simulink model "IOT_Charger"  (R2024b)
settings: Solver=ode23tb  StartTime=0.0  StopTime=1  RelTol=1e-3  EnableMultiTasking=on
PreLoadFcn:
  | % Data of Solar Panel
  | %5000[W]/130[W]
  | % Total power generated by solar panel reaches 5[KW].
  | % each solar panel generates power 130[kW].
  | V = [0    40 80 120 160 180 200 217 240 260 280];
  | I = 5000/130*[0.68 0.675 0.67 0.665 0.660 0.655 0.640 0.6 0.48 0.28 0];
  | 
  | %subplot(211);plot(V,I);xlabel('Voltage[V]');ylabel('Current[a]')
  | %subplot(212);plot(V.*I);title('Power[W]')
  | 
  | % Sample Time[s]
  | Ts =5e-6;
  | 
  | 
  | %MPPT + PV Control
  | % PI control pamameter of Voltage control(Outer loop)
  | Kp_V = 50e-3;
  | Ki_V = 10;
  | 
  | % PI Control pamameter of Current control(Inner loop)
  | Kp_I = 25e-3;
  | Ki_I = 10;
  | 
  | % Utility Interconnection Control
  | % PI Control pamameter of Voltage control(Outer loop)
  | Kp_V2 = 0.01;
  | Ki_V2 = 25;
  | 
  | % PI control pamameter of Current control(Inner loop)
  | Kp_I2 = 0.01;
  | Ki_I2 = 25;
  | 
  | 
  | % Difference of voltege using in MPPT
  | dV = 0.5;
  | 
  | % Battery Control
  | % PI Control pamameter of Voltage control(Outer loop)
  | Kp_VB = 0.4;
  | Ki_VB = 2;
  | 
  | % PI control pamameter of Current control(Inner loop)
  | Kp_IB = 0.1;
  | Ki_IB = 0.5;
undefined symbols (not defined in the file): Ion, Lithium, sigbuilder_block
libraries: spsBreakerLib x120, spsSeriesRLCBranchLib x72, spsBatteryLib x43, spsIdealSwitchLib x29, spsVoltageMeasurementLib x25, spsMosfetLib x19, slpidlib x17, spsSeriesRLCLoadLib x12, spsPWMGeneratorDCDCLib x11, spsCurrentMeasurementLib x10, spsDiodeLib x6, spsPWMGenerator2LevelLib x5
(part 4 of 6)

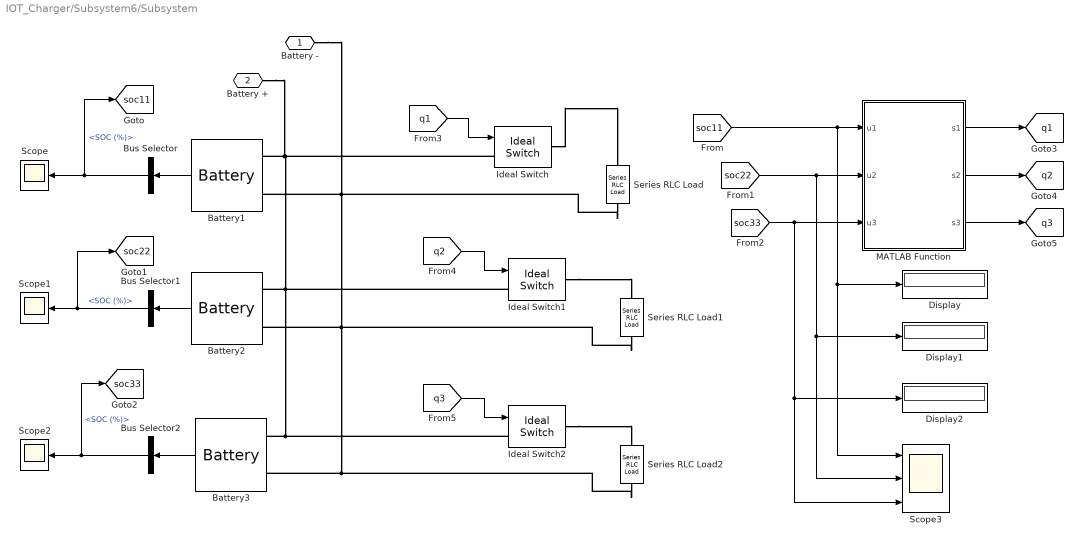
== system IOT_Charger/Subsystem6/Subsystem ==
  Battery1 : spsBatteryLib/Battery  BatType=Lithium-Ion  NomV=3.6  NomQ=4  SOC=100  Batt_Tr=1  PresetModel=on  MaxQ=4  MinV=2.7  FullV=4.1904  Dis_rate=1.7391  R=0.009  Normal_OP=3.6174  expZone="[3.8894     0.19652]"
  Battery2 : spsBatteryLib/Battery  BatType=Lithium-Ion  NomV=3.6  NomQ=4  SOC=60  Batt_Tr=1  PresetModel=on  MaxQ=4  MinV=2.7  FullV=4.1904  Dis_rate=1.7391  R=0.009  Normal_OP=3.6174  expZone="[3.8894     0.19652]"
  Battery3 : spsBatteryLib/Battery  BatType=Lithium-Ion  NomV=3.6  NomQ=4  SOC=30  Batt_Tr=1  PresetModel=on  MaxQ=4  MinV=2.7  FullV=4.1904  Dis_rate=1.7391  R=0.009  Normal_OP=3.6174  expZone="[3.8894     0.19652]"
  Bus Selector : BusSelector  OutputSignals=SOC (%)
  Bus Selector1 : BusSelector  OutputSignals=SOC (%)
  Bus Selector2 : BusSelector  OutputSignals=SOC (%)
  Display : Display
  Display1 : Display
  Display2 : Display
  Ideal Switch : spsIdealSwitchLib/Ideal Switch  Ron=0.001  Lon=0  IC=0  Rs=1e5  Cs=inf  Measurements=off
  Ideal Switch1 : spsIdealSwitchLib/Ideal Switch  Ron=0.001  Lon=0  IC=0  Rs=1e5  Cs=inf  Measurements=off
  Ideal Switch2 : spsIdealSwitchLib/Ideal Switch  Ron=0.001  Lon=0  IC=0  Rs=1e5  Cs=inf  Measurements=off
  MATLAB Function : MATLAB Function  TreatAsAtomicUnit=on
  Scope : Scope
  Scope1 : Scope
  Scope2 : Scope
  Scope3 : Scope  NumInputPorts=3
  Series RLC Load : spsSeriesRLCLoadLib/Series RLC Load  LConnTagsString=a  RConnTagsString=__new0  NominalVoltage=1000  NominalFrequency=60  ActivePower=10e3  InductivePower=0  CapacitivePower=0  Setx0=off  InitialVoltage=0  SetiL0=off  InitialCurrent=0  Measurements=None  LoadType=constant Z
  Series RLC Load1 : spsSeriesRLCLoadLib/Series RLC Load  LConnTagsString=a  RConnTagsString=__new0  NominalVoltage=1000  NominalFrequency=60  ActivePower=10e3  InductivePower=0  CapacitivePower=0  Setx0=off  InitialVoltage=0  SetiL0=off  InitialCurrent=0  Measurements=None  LoadType=constant Z
  Series RLC Load2 : spsSeriesRLCLoadLib/Series RLC Load  LConnTagsString=a  RConnTagsString=__new0  NominalVoltage=1000  NominalFrequency=60  ActivePower=10e3  InductivePower=0  CapacitivePower=0  Setx0=off  InitialVoltage=0  SetiL0=off  InitialCurrent=0  Measurements=None  LoadType=constant Z
  Battery - : PMIOPort  Side=Left
  Battery + : PMIOPort  Port=2  Side=Left
  tag scope: q1=global, q2=global, q3=global, soc11=global, soc22=global, soc33=global
  wires:
  Battery2/1 -> Bus Selector1/1
  Bus Selector/1 -> [soc11], Scope/1  "<SOC (%)>"
  [q3] -> Ideal Switch2/1
  Bus Selector2/1 -> [soc33], Scope2/1  "<SOC (%)>"
  Bus Selector1/1 -> [soc22], Scope1/1  "<SOC (%)>"
  Battery3/1 -> Bus Selector2/1
  [soc22] -> MATLAB Function/2(u2), Display1/1, Scope3/2
  [soc11] -> Display/1, Scope3/1, MATLAB Function/1(u1)
  Battery1/1 -> Bus Selector/1
  [soc33] -> Display2/1, Scope3/3, MATLAB Function/3(u3)
  MATLAB Function/2(s2) -> [q2]
  MATLAB Function/3(s3) -> [q3]
  MATLAB Function/1(s1) -> [q1]
  [q1] -> Ideal Switch/1
  [q2] -> Ideal Switch1/1
  connections:
  Series RLC Load/RConn1 -- Battery3/LConn2 -- Series RLC Load2/RConn1 -- Battery2/LConn2 -- Series RLC Load1/RConn1 -- Battery -/RConn1 -- Battery1/LConn2
  Ideal Switch1/RConn1 -- Series RLC Load1/LConn1
  Ideal Switch2/RConn1 -- Series RLC Load2/LConn1
  Ideal Switch/RConn1 -- Series RLC Load/LConn1
  Ideal Switch/LConn1 -- Battery +/RConn1 -- Battery1/LConn1 -- Battery3/LConn1 -- Ideal Switch2/LConn1 -- Battery2/LConn1 -- Ideal Switch1/LConn1

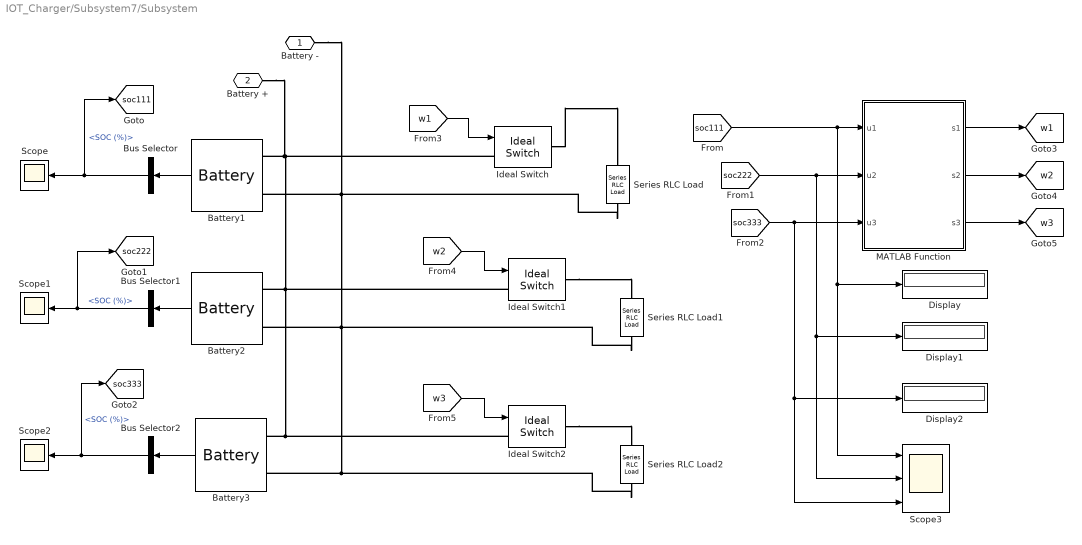
== system IOT_Charger/Subsystem7/Subsystem ==
  Battery1 : spsBatteryLib/Battery  BatType=Lithium-Ion  NomV=3.6  NomQ=4  SOC=100  Batt_Tr=1  PresetModel=on  MaxQ=4  MinV=2.7  FullV=4.1904  Dis_rate=1.7391  R=0.009  Normal_OP=3.6174  expZone="[3.8894     0.19652]"
  Battery2 : spsBatteryLib/Battery  BatType=Lithium-Ion  NomV=3.6  NomQ=4  SOC=60  Batt_Tr=1  PresetModel=on  MaxQ=4  MinV=2.7  FullV=4.1904  Dis_rate=1.7391  R=0.009  Normal_OP=3.6174  expZone="[3.8894     0.19652]"
  Battery3 : spsBatteryLib/Battery  BatType=Lithium-Ion  NomV=3.6  NomQ=4  SOC=30  Batt_Tr=1  PresetModel=on  MaxQ=4  MinV=2.7  FullV=4.1904  Dis_rate=1.7391  R=0.009  Normal_OP=3.6174  expZone="[3.8894     0.19652]"
  Bus Selector : BusSelector  OutputSignals=SOC (%)
  Bus Selector1 : BusSelector  OutputSignals=SOC (%)
  Bus Selector2 : BusSelector  OutputSignals=SOC (%)
  Display : Display
  Display1 : Display
  Display2 : Display
  Ideal Switch : spsIdealSwitchLib/Ideal Switch  Ron=0.001  Lon=0  IC=0  Rs=1e5  Cs=inf  Measurements=off
  Ideal Switch1 : spsIdealSwitchLib/Ideal Switch  Ron=0.001  Lon=0  IC=0  Rs=1e5  Cs=inf  Measurements=off
  Ideal Switch2 : spsIdealSwitchLib/Ideal Switch  Ron=0.001  Lon=0  IC=0  Rs=1e5  Cs=inf  Measurements=off
  MATLAB Function : MATLAB Function  TreatAsAtomicUnit=on
  Scope : Scope
  Scope1 : Scope
  Scope2 : Scope
  Scope3 : Scope  NumInputPorts=3
  Series RLC Load : spsSeriesRLCLoadLib/Series RLC Load  LConnTagsString=a  RConnTagsString=__new0  NominalVoltage=1000  NominalFrequency=60  ActivePower=10e3  InductivePower=0  CapacitivePower=0  Setx0=off  InitialVoltage=0  SetiL0=off  InitialCurrent=0  Measurements=None  LoadType=constant Z
  Series RLC Load1 : spsSeriesRLCLoadLib/Series RLC Load  LConnTagsString=a  RConnTagsString=__new0  NominalVoltage=1000  NominalFrequency=60  ActivePower=10e3  InductivePower=0  CapacitivePower=0  Setx0=off  InitialVoltage=0  SetiL0=off  InitialCurrent=0  Measurements=None  LoadType=constant Z
  Series RLC Load2 : spsSeriesRLCLoadLib/Series RLC Load  LConnTagsString=a  RConnTagsString=__new0  NominalVoltage=1000  NominalFrequency=60  ActivePower=10e3  InductivePower=0  CapacitivePower=0  Setx0=off  InitialVoltage=0  SetiL0=off  InitialCurrent=0  Measurements=None  LoadType=constant Z
  Battery - : PMIOPort  Side=Left
  Battery + : PMIOPort  Port=2  Side=Left
  tag scope: soc111=global, soc222=global, soc333=global, w1=global, w2=global, w3=global
  wires:
  Battery2/1 -> Bus Selector1/1
  Bus Selector/1 -> [soc111], Scope/1  "<SOC (%)>"
  [w3] -> Ideal Switch2/1
  Bus Selector2/1 -> [soc333], Scope2/1  "<SOC (%)>"
  Bus Selector1/1 -> [soc222], Scope1/1  "<SOC (%)>"
  Battery3/1 -> Bus Selector2/1
  [soc222] -> MATLAB Function/2(u2), Display1/1, Scope3/2
  [soc111] -> Display/1, Scope3/1, MATLAB Function/1(u1)
  Battery1/1 -> Bus Selector/1
  [soc333] -> Display2/1, Scope3/3, MATLAB Function/3(u3)
  MATLAB Function/2(s2) -> [w2]
  MATLAB Function/3(s3) -> [w3]
  MATLAB Function/1(s1) -> [w1]
  [w1] -> Ideal Switch/1
  [w2] -> Ideal Switch1/1
  connections:
  Series RLC Load/RConn1 -- Battery3/LConn2 -- Series RLC Load2/RConn1 -- Battery2/LConn2 -- Series RLC Load1/RConn1 -- Battery -/RConn1 -- Battery1/LConn2
  Ideal Switch1/RConn1 -- Series RLC Load1/LConn1
  Ideal Switch2/RConn1 -- Series RLC Load2/LConn1
  Ideal Switch/RConn1 -- Series RLC Load/LConn1
  Ideal Switch/LConn1 -- Battery +/RConn1 -- Battery1/LConn1 -- Battery3/LConn1 -- Ideal Switch2/LConn1 -- Battery2/LConn1 -- Ideal Switch1/LConn1

== system IOT_Charger/Vechicle BMS Monitoring/BMS Discharge ==
  Terminal voltage : Inport
  Temperature : Inport  Port=2
  Current : Inport  Port=3
  Constant : Constant  Value=0
  Function logic block : Subsystem
  Switch : Switch  Criteria=u2 ~= 0  SaturateOnIntegerOverflow=off  InputSameDT=off
  Discharge current : Outport
  wires:
  Terminal voltage/1 -> Function logic block/1(Terminal voltage)
  Current/1 -> Switch/3, Function logic block/2(Current)
  Temperature/1 -> Function logic block/3(Temperature)
  Function logic block/1(Discharge Terget) -> Switch/2
  Constant/1 -> Switch/1
  Switch/1 -> Discharge current/1

== system IOT_Charger/Vechicle BMS Monitoring1/BMS Discharge ==
  Terminal voltage : Inport
  Temperature : Inport  Port=2
  Current : Inport  Port=3
  Constant : Constant  Value=0
  Function logic block : Subsystem
  Switch : Switch  Criteria=u2 ~= 0  SaturateOnIntegerOverflow=off  InputSameDT=off
  Discharge current : Outport
  wires:
  Terminal voltage/1 -> Function logic block/1(Terminal voltage)
  Current/1 -> Switch/3, Function logic block/2(Current)
  Temperature/1 -> Function logic block/3(Temperature)
  Function logic block/1(Discharge Terget) -> Switch/2
  Constant/1 -> Switch/1
  Switch/1 -> Discharge current/1

== system IOT_Charger/Vechicle BMS Monitoring2/BMS Discharge ==
  Terminal voltage : Inport
  Temperature : Inport  Port=2
  Current : Inport  Port=3
  Constant : Constant  Value=0
  Function logic block : Subsystem
  Switch : Switch  Criteria=u2 ~= 0  SaturateOnIntegerOverflow=off  InputSameDT=off
  Discharge current : Outport
  wires:
  Terminal voltage/1 -> Function logic block/1(Terminal voltage)
  Current/1 -> Switch/3, Function logic block/2(Current)
  Temperature/1 -> Function logic block/3(Temperature)
  Function logic block/1(Discharge Terget) -> Switch/2
  Constant/1 -> Switch/1
  Switch/1 -> Discharge current/1

== system IOT_Charger/Vechicle BMS Monitoring3/BMS Discharge ==
  Terminal voltage : Inport
  Temperature : Inport  Port=2
  Current : Inport  Port=3
  Constant : Constant  Value=0
  Function logic block : Subsystem
  Switch : Switch  Criteria=u2 ~= 0  SaturateOnIntegerOverflow=off  InputSameDT=off
  Discharge current : Outport
  wires:
  Terminal voltage/1 -> Function logic block/1(Terminal voltage)
  Current/1 -> Switch/3, Function logic block/2(Current)
  Temperature/1 -> Function logic block/3(Temperature)
  Function logic block/1(Discharge Terget) -> Switch/2
  Constant/1 -> Switch/1
  Switch/1 -> Discharge current/1

== system IOT_Charger/Fast charging controller/Fast charging Switching controller/g1 ==
  Constant1 : Constant  Value=0
  Constant2 : Constant
  Display2 : Display
  Display3 : Display
  Switch : Switch  Threshold=150  SaturateOnIntegerOverflow=off  InputSameDT=off
  tag scope: gg1=global
  wires:
  [FS] -> Display3/1, Switch/2
  Switch/1 -> Display2/1, [gg1]
  Constant1/1 -> Switch/3
  Constant2/1 -> Switch/1

== system IOT_Charger/Fast charging controller/Fast charging Switching controller/g2 ==
  Constant1 : Constant  Value=0
  Constant2 : Constant
  Display2 : Display
  Display3 : Display
  Switch : Switch  Threshold=150  SaturateOnIntegerOverflow=off  InputSameDT=off
  tag scope: gg2=global
  wires:
  [FS] -> Display3/1, Switch/2
  Switch/1 -> Display2/1, [gg2]
  Constant1/1 -> Switch/3
  Constant2/1 -> Switch/1

== system IOT_Charger/Fast charging controller/Fast charging Switching controller/g3 ==
  Constant1 : Constant  Value=0
  Constant2 : Constant
  Display2 : Display
  Display3 : Display
  Switch : Switch  Threshold=150  SaturateOnIntegerOverflow=off  InputSameDT=off
  tag scope: gg3=global
  wires:
  [FS] -> Display3/1, Switch/2
  Switch/1 -> Display2/1, [gg3]
  Constant1/1 -> Switch/3
  Constant2/1 -> Switch/1

== system IOT_Charger/Fast charging controller/Fast charging Switching controller/g4 ==
  Constant1 : Constant  Value=0
  Constant2 : Constant
  Display2 : Display
  Display3 : Display
  Switch : Switch  Threshold=150  SaturateOnIntegerOverflow=off  InputSameDT=off
  tag scope: gg4=global
  wires:
  [FS] -> Display3/1, Switch/2
  Switch/1 -> Display2/1, [gg4]
  Constant1/1 -> Switch/3
  Constant2/1 -> Switch/1

== system IOT_Charger/Grid/Wall charger Connection Box/Battery Switching Control ==
  Control : Inport
  Ideal Switch{,1,3..4} (4 alike) : spsIdealSwitchLib/Ideal Switch  Ron=0.001  Lon=0  IC=0  Rs=1e5  Cs=inf  Measurements=off
  NOT : Logic  Operator=NOT  IconShape=distinctive  AllPortsSameDT=off  OutDataTypeStr=boolean
  discharge + : PMIOPort  Side=Left
  discharge - : PMIOPort  Port=2  Side=Left
  charge + : PMIOPort  Port=3  Side=Left
  charge - : PMIOPort  Port=4  Side=Left
  battery + : PMIOPort  Port=5  Side=Right
  battery - : PMIOPort  Port=6  Side=Right
  wires:
  Control/1 -> NOT/1, Ideal Switch1/1, Ideal Switch/1
  NOT/1 -> Ideal Switch4/1, Ideal Switch3/1
  connections:
  charge -/RConn1 -- Ideal Switch4/RConn1
  discharge +/RConn1 -- Ideal Switch/RConn1
  Ideal Switch1/LConn1 -- battery -/RConn1 -- Ideal Switch4/LConn1
  discharge -/RConn1 -- Ideal Switch1/RConn1
  Ideal Switch/LConn1 -- battery +/RConn1 -- Ideal Switch3/LConn1
  charge +/RConn1 -- Ideal Switch3/RConn1

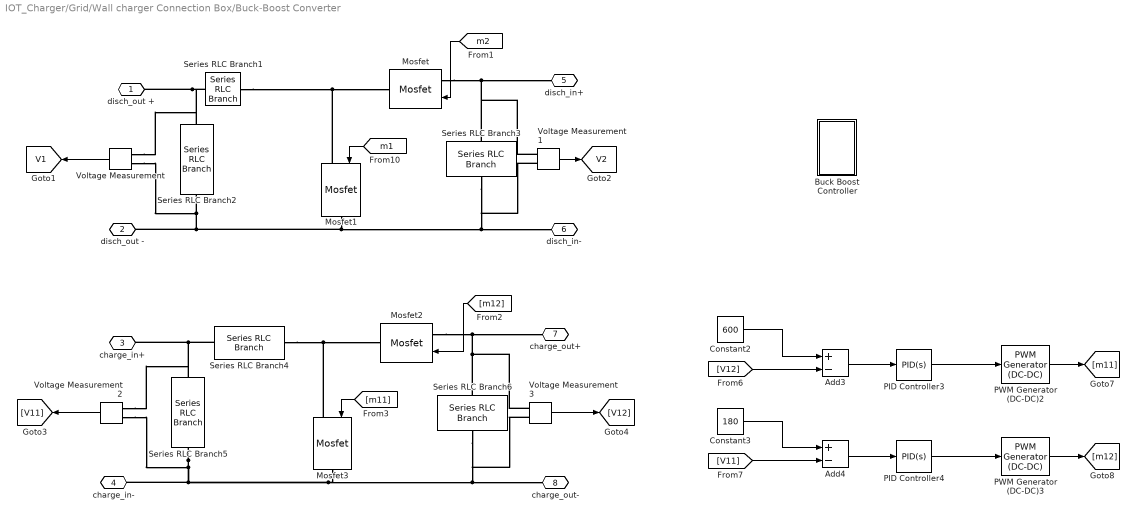
== system IOT_Charger/Grid/Wall charger Connection Box/Buck-Boost Converter ==
  Add3 : Sum  Inputs=+-
  Add4 : Sum  Inputs=+-
  Buck Boost Controller : Subsystem
  Constant2 : Constant  Value=600
  Constant3 : Constant  Value=180
  Mosfet{,1..3} (4 alike) : spsMosfetLib/Mosfet  Ron=0.1  Lon=0  Rd=0.01  Vfd=0  IC=0  Rs=1e5  Cs=inf  Measurements=off
  PID Controller3 : slpidlib/PID Controller  Controller=PID  Form=Parallel  TimeDomain=Continuous-time  UseExternalTs=off  SampleTime=-1  IntegratorMethod=Forward Euler  FilterMethod=Forward Euler  ControllerParametersSource=internal  P=0  I=7  UseKiTs=off  D=0  UseExternalDerivativeSource=off  N=100  UseFilter=on  TunerSelectOption=Transfer Function Based (PID Tuner App)  InitialConditionSource=internal  InitialConditionForIntegrator=0  InitialConditionForFilter=0  DifferentiatorICPrevScaledInput=0  ExternalReset=none  TrackingMode=off  Kt=1  LimitOutput=off  SatLimitsSource=internal  UpperSaturationLimit=inf  LowerSaturationLimit=-inf  LinearizeAsGain=on  AntiWindupMode=none  Kb=1  LimitIntegrator=off  UpperIntegratorSaturationLimit=inf  LowerIntegratorSaturationLimit=-inf  POutMin=[]  POutMax=[]  IOutMin=[]  IOutMax=[]  DOutMin=[]  DOutMax=[]  NOutMin=[]  NOutMax=[]  SumOutMin=[]  SumOutMax=[]  SaturationOutMin=[]  SaturationOutMax=[]  PParamMin=[]  PParamMax=[]  IParamMin=[]  IParamMax=[]  DParamMin=[]  DParamMax=[]  NParamMin=[]  NParamMax=[]  KbParamMin=[]  KbParamMax=[]  KtParamMin=[]  KtParamMax=[]  KbOutMin=[]  KbOutMax=[]  KtOutMin=[]  KtOutMax=[]  IntegratorOutMin=[]  IntegratorOutMax=[]  FilterOutMin=[]  FilterOutMax=[]  SumI1OutMin=[]  SumI1OutMax=[]  SumI2OutMin=[]  SumI2OutMax=[]  SumI3OutMin=[]  SumI3OutMax=[]  SumI4OutMin=[]  SumI4OutMax=[]  SumDOutMin=[]  SumDOutMax=[]  DifferentiatorOutMin=[]  DifferentiatorOutMax=[]  FilterDiffOutCoefMin=[]  FilterDiffOutCoefMax=[]  ReciprocalOutMin=[]  ReciprocalOutMax=[]  SumDenOutMin=[]  SumDenOutMax=[]  SumNumOutMin=[]  SumNumOutMax=[]  DivideOutMin=[]  DivideOutMax=[]  UdiffTsProdOutMin=[]  UdiffTsProdOutMax=[]  NTsProdOutMin=[]  NTsProdOutMax=[]  UintegralTsProdOutMin=[]  UintegralTsProdOutMax=[]  UngainTsProdOutMin=[]  UngainTsProdOutMax=[]  ClampingZeroOutDataTypeStr=Inherit: Inherit via back propagation  ClampingZeroOutMin=[]  ClampingZeroOutMax=[]  FilterDenConstantOutDataTypeStr=Inherit: Inherit via back propagation  FilterDenConstantOutMin=[]  FilterDenConstantOutMax=[]  PCopyOutDataTypeStr=Inherit: Inherit via back propagation  PCopyOutMin=[]  PCopyOutMax=[]  NCopyOutDataTypeStr=Inherit: Inherit via back propagation  NCopyOutMin=[]  NCopyOutMax=[]  IntegratorContinuousStateAttributes=''  IntegratorStateMustResolveToSignalObject=off  IntegratorRTWStateStorageClass=Auto  FilterContinuousStateAttributes=''  FilterStateMustResolveToSignalObject=off  FilterRTWStateStorageClass=Auto  ParallelPVariant=InternalParameters  IdealPVariant=Disabled  IVariant=InternalParameters  DVariant=InternalParameters  IntegratorVariant=Continuous  SatVariant=Disabled  AWVariant=Passthrough  PCopyVariant=Disabled  TRVariant=Disabled  FdbkBlocksVariant=Forward  IdealPFdbkVariant=Disabled  SatFdbkVariant=Disabled  DerivativeFilterVariant=ContFilter  NVariant=InternalParameters  NCopyVariant=Disabled  FilterICVariant=InternalICsFilter  IntegratorICVariant=InternalICs  ExternalResetVariant=Disabled  TRSumVariant=Passthrough  SumFdbkVariant=Disabled  SumVariant=Sum_PID  TsampFilterVariant=InternalTs  TsampNgainVariant=Passthrough  TsampIntegralVariant=Disabled_SignalSpec  ExternalSaturationOutDataTypeStr=Inherit: Same as second input  DerivativeSourceVariant=ErrorSignal  PreIntVariant=InternalPreInt
  PID Controller4 : slpidlib/PID Controller  Controller=PID  Form=Parallel  TimeDomain=Continuous-time  UseExternalTs=off  SampleTime=-1  IntegratorMethod=Forward Euler  FilterMethod=Forward Euler  ControllerParametersSource=internal  P=0  I=7  UseKiTs=off  D=0  UseExternalDerivativeSource=off  N=100  UseFilter=on  TunerSelectOption=Transfer Function Based (PID Tuner App)  InitialConditionSource=internal  InitialConditionForIntegrator=0  InitialConditionForFilter=0  DifferentiatorICPrevScaledInput=0  ExternalReset=none  TrackingMode=off  Kt=1  LimitOutput=off  SatLimitsSource=internal  UpperSaturationLimit=inf  LowerSaturationLimit=-inf  LinearizeAsGain=on  AntiWindupMode=none  Kb=1  LimitIntegrator=off  UpperIntegratorSaturationLimit=inf  LowerIntegratorSaturationLimit=-inf  POutMin=[]  POutMax=[]  IOutMin=[]  IOutMax=[]  DOutMin=[]  DOutMax=[]  NOutMin=[]  NOutMax=[]  SumOutMin=[]  SumOutMax=[]  SaturationOutMin=[]  SaturationOutMax=[]  PParamMin=[]  PParamMax=[]  IParamMin=[]  IParamMax=[]  DParamMin=[]  DParamMax=[]  NParamMin=[]  NParamMax=[]  KbParamMin=[]  KbParamMax=[]  KtParamMin=[]  KtParamMax=[]  KbOutMin=[]  KbOutMax=[]  KtOutMin=[]  KtOutMax=[]  IntegratorOutMin=[]  IntegratorOutMax=[]  FilterOutMin=[]  FilterOutMax=[]  SumI1OutMin=[]  SumI1OutMax=[]  SumI2OutMin=[]  SumI2OutMax=[]  SumI3OutMin=[]  SumI3OutMax=[]  SumI4OutMin=[]  SumI4OutMax=[]  SumDOutMin=[]  SumDOutMax=[]  DifferentiatorOutMin=[]  DifferentiatorOutMax=[]  FilterDiffOutCoefMin=[]  FilterDiffOutCoefMax=[]  ReciprocalOutMin=[]  ReciprocalOutMax=[]  SumDenOutMin=[]  SumDenOutMax=[]  SumNumOutMin=[]  SumNumOutMax=[]  DivideOutMin=[]  DivideOutMax=[]  UdiffTsProdOutMin=[]  UdiffTsProdOutMax=[]  NTsProdOutMin=[]  NTsProdOutMax=[]  UintegralTsProdOutMin=[]  UintegralTsProdOutMax=[]  UngainTsProdOutMin=[]  UngainTsProdOutMax=[]  ClampingZeroOutDataTypeStr=Inherit: Inherit via back propagation  ClampingZeroOutMin=[]  ClampingZeroOutMax=[]  FilterDenConstantOutDataTypeStr=Inherit: Inherit via back propagation  FilterDenConstantOutMin=[]  FilterDenConstantOutMax=[]  PCopyOutDataTypeStr=Inherit: Inherit via back propagation  PCopyOutMin=[]  PCopyOutMax=[]  NCopyOutDataTypeStr=Inherit: Inherit via back propagation  NCopyOutMin=[]  NCopyOutMax=[]  IntegratorContinuousStateAttributes=''  IntegratorStateMustResolveToSignalObject=off  IntegratorRTWStateStorageClass=Auto  FilterContinuousStateAttributes=''  FilterStateMustResolveToSignalObject=off  FilterRTWStateStorageClass=Auto  ParallelPVariant=InternalParameters  IdealPVariant=Disabled  IVariant=InternalParameters  DVariant=InternalParameters  IntegratorVariant=Continuous  SatVariant=Disabled  AWVariant=Passthrough  PCopyVariant=Disabled  TRVariant=Disabled  FdbkBlocksVariant=Forward  IdealPFdbkVariant=Disabled  SatFdbkVariant=Disabled  DerivativeFilterVariant=ContFilter  NVariant=InternalParameters  NCopyVariant=Disabled  FilterICVariant=InternalICsFilter  IntegratorICVariant=InternalICs  ExternalResetVariant=Disabled  TRSumVariant=Passthrough  SumFdbkVariant=Disabled  SumVariant=Sum_PID  TsampFilterVariant=InternalTs  TsampNgainVariant=Passthrough  TsampIntegralVariant=Disabled_SignalSpec  ExternalSaturationOutDataTypeStr=Inherit: Same as second input  DerivativeSourceVariant=ErrorSignal  PreIntVariant=InternalPreInt
  PWM Generator (DC-DC)2 : spsPWMGeneratorDCDCLib/PWM Generator (DC-DC)  Fsw=5000  Ts=0
  PWM Generator (DC-DC)3 : spsPWMGeneratorDCDCLib/PWM Generator (DC-DC)  Fsw=5000  Ts=0
  Series RLC Branch1 : spsSeriesRLCBranchLib/Series RLC Branch  LConnTagsString=__new0  RConnTagsString=__new0  BranchType=L  Resistance=1  Inductance=1e-3  SetiL0=off  InitialCurrent=0  Capacitance=1e-6  Setx0=off  InitialVoltage=0  Measurements=None
  Series RLC Branch{2..3,5..6} (4 alike) : spsSeriesRLCBranchLib/Series RLC Branch  LConnTagsString=__new0  RConnTagsString=__new0  BranchType=RC  Resistance=0.0001  Inductance=1e-3  SetiL0=off  InitialCurrent=0  Capacitance=1000e-6  Setx0=off  InitialVoltage=0  Measurements=None
  Series RLC Branch4 : spsSeriesRLCBranchLib/Series RLC Branch  LConnTagsString=__new0  RConnTagsString=__new0  BranchType=L  Resistance=100e3  Inductance=1e-3  SetiL0=off  InitialCurrent=0  Capacitance=1e-6  Setx0=off  InitialVoltage=0  Measurements=None
  Voltage Measurement{,1..3} (4 alike) : spsVoltageMeasurementLib/Voltage Measurement  PhasorSimulation=off  OutputType=Complex  PSBequivalent=0
  disch_out + : PMIOPort  Side=Left
  disch_out - : PMIOPort  Port=2  Side=Left
  charge_in+ : PMIOPort  Port=3  Side=Left
  charge_in- : PMIOPort  Port=4  Side=Left
  disch_in+ : PMIOPort  Port=5  Side=Right
  disch_in- : PMIOPort  Port=6  Side=Right
  charge_out+ : PMIOPort  Port=7  Side=Right
  charge_out- : PMIOPort  Port=8  Side=Right
  tag scope: V1=global, V2=global
  wires:
  Voltage Measurement1/1 -> [V2]
  Voltage Measurement/1 -> [V1]
  PWM Generator (DC-DC)2/1 -> [m11]
  [V11] -> Add4/2
  Add3/1 -> PID Controller3/1
  Voltage Measurement3/1 -> [V12]
  PID Controller4/1 -> PWM Generator (DC-DC)3/1
  PID Controller3/1 -> PWM Generator (DC-DC)2/1
  Add4/1 -> PID Controller4/1
  [m11] -> Mosfet3/1
  Voltage Measurement2/1 -> [V11]
  PWM Generator (DC-DC)3/1 -> [m12]
  [m12] -> Mosfet2/1
  Constant3/1 -> Add4/1
  Constant2/1 -> Add3/1
  [V12] -> Add3/2
  [m1] -> Mosfet1/1
  [m2] -> Mosfet/1
  connections:
  Series RLC Branch5/RConn1 -- charge_in-/RConn1 -- charge_out-/RConn1 -- Voltage Measurement3/LConn2 -- Series RLC Branch6/RConn1 -- Mosfet3/RConn1 -- Voltage Measurement2/LConn2
  Mosfet1/RConn1 -- disch_in-/RConn1 -- Voltage Measurement1/LConn2 -- Series RLC Branch3/RConn1 -- disch_out -/RConn1 -- Voltage Measurement/LConn2 -- Series RLC Branch2/RConn1
  Mosfet/LConn1 -- disch_in+/RConn1 -- Voltage Measurement1/LConn1 -- Series RLC Branch3/LConn1
  Series RLC Branch4/LConn1 -- charge_in+/RConn1 -- Voltage Measurement2/LConn1 -- Series RLC Branch5/LConn1
  Series RLC Branch1/LConn1 -- Voltage Measurement/LConn1 -- Series RLC Branch2/LConn1 -- disch_out +/RConn1
  Series RLC Branch6/LConn1 -- Voltage Measurement3/LConn1 -- charge_out+/RConn1 -- Mosfet2/LConn1
  Mosfet1/LConn1 -- Series RLC Branch1/RConn1 -- Mosfet/RConn1
  Series RLC Branch4/RConn1 -- Mosfet3/LConn1 -- Mosfet2/RConn1

== system IOT_Charger/Grid/Wall charger Connection Box/Connection Control ==
  Control : Inport
  Ideal Switch{,1..5} (6 alike) : spsIdealSwitchLib/Ideal Switch  Ron=0.001  Lon=0  IC=0  Rs=1e5  Cs=inf  Measurements=off
  NOT : Logic  Operator=NOT  IconShape=distinctive  AllPortsSameDT=off  OutDataTypeStr=boolean
  Grid R : PMIOPort  Side=Left
  Grid Y : PMIOPort  Port=2  Side=Left
  Grid B : PMIOPort  Port=3  Side=Left
  Discharge R : PMIOPort  Port=4  Side=Right
  Discharge Y : PMIOPort  Port=5  Side=Right
  Discharge B : PMIOPort  Port=6  Side=Right
  charge R : PMIOPort  Port=7  Side=Right
  charge Y : PMIOPort  Port=8  Side=Right
  charge B : PMIOPort  Port=9  Side=Right
  wires:
  Control/1 -> NOT/1, Ideal Switch2/1, Ideal Switch1/1, Ideal Switch/1
  NOT/1 -> Ideal Switch5/1, Ideal Switch4/1, Ideal Switch3/1
  connections:
  Ideal Switch2/RConn1 -- Grid B/RConn1 -- Ideal Switch5/RConn1
  Discharge R/RConn1 -- Ideal Switch/LConn1
  Discharge B/RConn1 -- Ideal Switch2/LConn1
  Ideal Switch/RConn1 -- Grid R/RConn1 -- Ideal Switch3/RConn1
  Ideal Switch1/RConn1 -- Grid Y/RConn1 -- Ideal Switch4/RConn1
  Ideal Switch4/LConn1 -- charge Y/RConn1
  Discharge Y/RConn1 -- Ideal Switch1/LConn1
  charge R/RConn1 -- Ideal Switch3/LConn1
  Ideal Switch5/LConn1 -- charge B/RConn1

== system IOT_Charger/Grid/Wall charger Connection Box/DC-AC // AC-DC Converter ==
  Controller : Subsystem
  Measurement1 : spsThreePhaseVIMeasurementLib/Three-Phase V-I Measurement  VoltageMeasurement=phase-to-ground  SetLabelV=on  LabelV=Vabc_inv  Vpu=off  VpuLL=off  CurrentMeasurement=yes  SetLabelI=on  LabelI=Iabc_inv  Ipu=off  Pbase=100e6  Vbase=500e3  OutputType=Complex  PhasorSimulation=off  PSBequivalent=0
  PWM Generator (2-Level) : spsPWMGenerator2LevelLib/PWM Generator (2-Level)  ModulatorType=Three-phase bridge (6 pulses)  ModulatorMode=Unsynchronized  Fc=4950  Pc=90  nF=27  MinMax="[ -1  1 ]"  SamplingTechnique=Natural  ModulatingSignals=off  m=0.8  Freq=60  Phase=0  Ts=2.02e-6  ShowCarrierOutport=off
  Parallel Connection control : Constant
  Series RLC Branch2 : spsSeriesRLCBranchLib/Series RLC Branch  LConnTagsString=__new0  RConnTagsString=__new0  BranchType=RC  Resistance=10e3  Inductance=1e-3  SetiL0=off  InitialCurrent=0  Capacitance=1000e-6  Setx0=off  InitialVoltage=0  Measurements=None
  Three-Phase Series RLC Branch : spsThreePhaseSeriesRLCBranchLib/Three-Phase Series RLC Branch  LConnTagsString=A|B|C  RConnTagsString=A|B|C  BranchType=RL  Resistance=0.004332  Inductance=0.0013789184  Capacitance=1e-6  Measurements=None
  Three-Phase Breaker : spsThreePhaseBreakerLib/Three-Phase Breaker  InitialState=open  SwitchA=on  SwitchB=on  SwitchC=on  SwitchTimes="[1/60  5/60]"  External=on  BreakerResistance=0.01  SnubberResistance=1e6  SnubberCapacitance=inf  Measurements=None
  Transformer near home1 : spsThreePhaseSeriesRLCLoadLib/Three-Phase Series RLC Load  LConnTagsString=A|B|C  Configuration=Delta  NominalVoltage=380  Vabc=[1e3 1e3 1e3]  Vabcp=[1e3 1e3 1e3]  NominalFrequency=50  UnbalancedPower=off  ActivePower=100  InductivePower=0  CapacitivePower=5000  Pabc=[10e3 9e3 11e3]  QLabc=[100 90 110]  QCabc=[100 90 110]  Pabcp=[10e3 9e3 11e3]  QLabcp=[100 90 110]  QCabcp=[100 90 110]  Measurements=None  LoadType=constant Z
  Universal Bridge : spsUniversalBridgeLib/Universal Bridge  Arms=3  SnubberResistance=1e5  SnubberCapacitance=inf  Device=IGBT / Diodes  Ron=1e-3  Lon=0  ForwardVoltages="[  0  0  ]"  ForwardVoltage=0  GTOparameters=[ 10e-6 , 20e-6 ]  IGBTparameters=[ 1e-6 , 2e-6 ]  Measurements=None  Measurements_2=None  converterType=Rectifier
  Universal Bridge1 : spsUniversalBridgeLib/Universal Bridge  Arms=3  SnubberResistance=1e5  SnubberCapacitance=inf  Device=Diodes  Ron=1e-3  Lon=0  ForwardVoltages="[  0  0  ]"  ForwardVoltage=0  GTOparameters=[ 10e-6 , 20e-6 ]  IGBTparameters=[ 1e-6 , 2e-6 ]  Measurements=None  Measurements_2=None  converterType=Rectifier
  Discharge_R : PMIOPort  Side=Left
  Discharge_Y : PMIOPort  Port=2  Side=Left
  Discharge_B : PMIOPort  Port=3  Side=Left
  charge_R : PMIOPort  Port=4  Side=Left
  charge_Y : PMIOPort  Port=5  Side=Left
  charge_B : PMIOPort  Port=6  Side=Left
  Discharge + : PMIOPort  Port=7  Side=Right
  Discharge - : PMIOPort  Port=8  Side=Right
  charge+ : PMIOPort  Port=9  Side=Right
  charge- : PMIOPort  Port=10  Side=Right
  wires:
  PWM Generator (2-Level)/1 -> Universal Bridge/1
  Parallel Connection control/1 -> Three-Phase Breaker/1
  [ref] -> PWM Generator (2-Level)/1
  connections:
  Universal Bridge1/LConn2 -- charge_Y/RConn1
  Universal Bridge1/LConn3 -- charge_B/RConn1
  Discharge_Y/RConn1 -- Three-Phase Breaker/RConn2
  Three-Phase Series RLC Branch/RConn1 -- Transformer near home1/LConn1 -- Measurement1/LConn1
  Measurement1/RConn2 -- Three-Phase Breaker/LConn2
  charge-/RConn1 -- Series RLC Branch2/RConn1 -- Universal Bridge1/RConn2
  Three-Phase Series RLC Branch/RConn3 -- Measurement1/LConn3 -- Transformer near home1/LConn3
  Discharge_B/RConn1 -- Three-Phase Breaker/RConn3
  Three-Phase Series RLC Branch/LConn2 -- Universal Bridge/LConn2
  Universal Bridge/LConn1 -- Three-Phase Series RLC Branch/LConn1
  Discharge -/RConn1 -- Universal Bridge/RConn2
  Universal Bridge/LConn3 -- Three-Phase Series RLC Branch/LConn3
  Three-Phase Series RLC Branch/RConn2 -- Measurement1/LConn2 -- Transformer near home1/LConn2
  Discharge +/RConn1 -- Universal Bridge/RConn1
  charge+/RConn1 -- Series RLC Branch2/LConn1 -- Universal Bridge1/RConn1
  Discharge_R/RConn1 -- Three-Phase Breaker/RConn1
  Measurement1/RConn1 -- Three-Phase Breaker/LConn1
  Measurement1/RConn3 -- Three-Phase Breaker/LConn3
  Universal Bridge1/LConn1 -- charge_R/RConn1

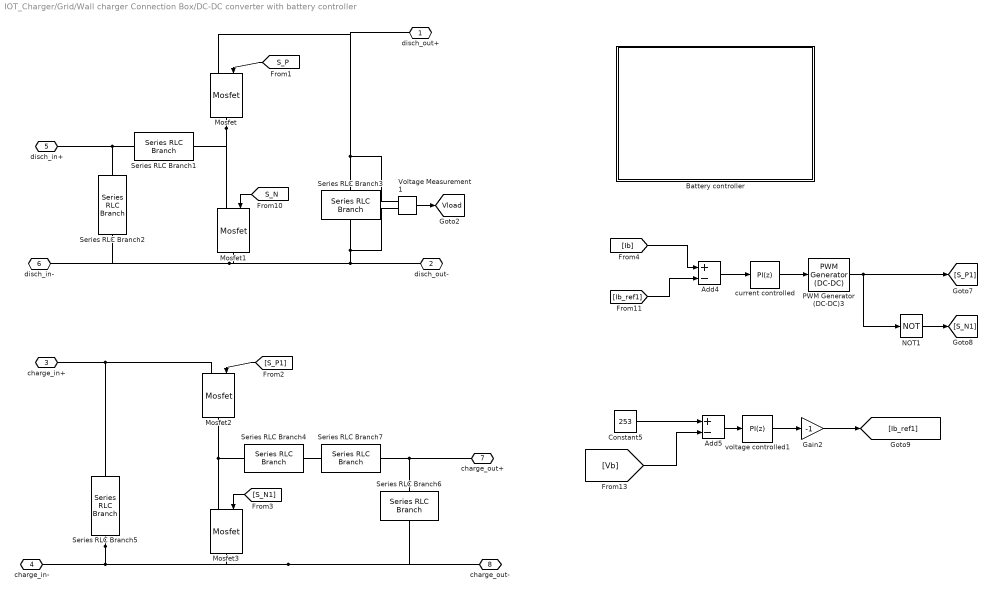
== system IOT_Charger/Grid/Wall charger Connection Box/DC-DC converter with battery controller ==
  Add4 : Sum  Inputs=+-
  Add5 : Sum  Inputs=+-
  Battery controller : Subsystem
  Constant5 : Constant  Value=253
  Gain2 : Gain  Gain=-1
  Mosfet{,1..3} (4 alike) : spsMosfetLib/Mosfet  Ron=0.1  Lon=0  Rd=0.01  Vfd=0  IC=0  Rs=1e5  Cs=inf  Measurements=off
  NOT1 : Logic  Operator=NOT  IconShape=distinctive  AllPortsSameDT=off  OutDataTypeStr=boolean
  PWM Generator (DC-DC)3 : spsPWMGeneratorDCDCLib/PWM Generator (DC-DC)  Fsw=10e3  Ts=5e-6
  Series RLC Branch1 : spsSeriesRLCBranchLib/Series RLC Branch  LConnTagsString=__new0  RConnTagsString=__new0  BranchType=RL  Resistance=1000  Inductance=5.76e-4  SetiL0=off  InitialCurrent=0  Capacitance=1e-6  Setx0=off  InitialVoltage=0  Measurements=None
  Series RLC Branch2 : spsSeriesRLCBranchLib/Series RLC Branch  LConnTagsString=__new0  RConnTagsString=__new0  BranchType=R  Resistance=10  Inductance=1e-3  SetiL0=off  InitialCurrent=0  Capacitance=1000e-6  Setx0=off  InitialVoltage=0  Measurements=None
  Series RLC Branch3 : spsSeriesRLCBranchLib/Series RLC Branch  LConnTagsString=__new0  RConnTagsString=__new0  BranchType=RC  Resistance=0.001  Inductance=1e-3  SetiL0=off  InitialCurrent=0  Capacitance=1000e-6  Setx0=off  InitialVoltage=0  Measurements=None
  Series RLC Branch4 : spsSeriesRLCBranchLib/Series RLC Branch  LConnTagsString=__new0  RConnTagsString=__new0  BranchType=RL  Resistance=0.05  Inductance=5.76e-4  SetiL0=off  InitialCurrent=0  Capacitance=1000e-6  Setx0=off  InitialVoltage=0  Measurements=None
  Series RLC Branch5 : spsSeriesRLCBranchLib/Series RLC Branch  LConnTagsString=__new0  RConnTagsString=__new0  BranchType=RC  Resistance=0.001  Inductance=1e-3  SetiL0=off  InitialCurrent=0  Capacitance=1000e-6  Setx0=off  InitialVoltage=0  Measurements=None
  Series RLC Branch6 : spsSeriesRLCBranchLib/Series RLC Branch  LConnTagsString=__new0  RConnTagsString=__new0  BranchType=RC  Resistance=1e-3  Inductance=1e-3  SetiL0=off  InitialCurrent=0  Capacitance=5600e-6  Setx0=off  InitialVoltage=0  Measurements=None
  Series RLC Branch7 : spsSeriesRLCBranchLib/Series RLC Branch  LConnTagsString=__new0  RConnTagsString=__new0  BranchType=R  Resistance=10  Inductance=1e-3  SetiL0=off  InitialCurrent=0  Capacitance=1000e-6  Setx0=off  InitialVoltage=0  Measurements=None
  Voltage Measurement1 : spsVoltageMeasurementLib/Voltage Measurement  PhasorSimulation=off  OutputType=Complex  PSBequivalent=0
  current controlled : slpidlib/PID Controller  Controller=PI  Form=Parallel  TimeDomain=Discrete-time  UseExternalTs=off  SampleTime=500e-6  IntegratorMethod=Forward Euler  FilterMethod=Forward Euler  ControllerParametersSource=internal  P=0.005  I=10  UseKiTs=off  D=0  UseExternalDerivativeSource=off  N=100  UseFilter=on  TunerSelectOption=Transfer Function Based (PID Tuner App)  InitialConditionSource=internal  InitialConditionForIntegrator=0.54  InitialConditionForFilter=0  DifferentiatorICPrevScaledInput=0  ExternalReset=none  TrackingMode=off  Kt=1  LimitOutput=on  SatLimitsSource=internal  UpperSaturationLimit=0.95  LowerSaturationLimit=0  LinearizeAsGain=on  AntiWindupMode=none  Kb=1  LimitIntegrator=off  UpperIntegratorSaturationLimit=inf  LowerIntegratorSaturationLimit=-inf  POutMin=[]  POutMax=[]  IOutMin=[]  IOutMax=[]  DOutMin=[]  DOutMax=[]  NOutMin=[]  NOutMax=[]  SumOutMin=[]  SumOutMax=[]  SaturationOutMin=[]  SaturationOutMax=[]  PParamMin=[]  PParamMax=[]  IParamMin=[]  IParamMax=[]  DParamMin=[]  DParamMax=[]  NParamMin=[]  NParamMax=[]  KbParamMin=[]  KbParamMax=[]  KtParamMin=[]  KtParamMax=[]  KbOutMin=[]  KbOutMax=[]  KtOutMin=[]  KtOutMax=[]  IntegratorOutMin=[]  IntegratorOutMax=[]  FilterOutMin=[]  FilterOutMax=[]  SumI1OutMin=[]  SumI1OutMax=[]  SumI2OutMin=[]  SumI2OutMax=[]  SumI3OutMin=[]  SumI3OutMax=[]  SumI4OutMin=[]  SumI4OutMax=[]  SumDOutMin=[]  SumDOutMax=[]  DifferentiatorOutMin=[]  DifferentiatorOutMax=[]  FilterDiffOutCoefMin=[]  FilterDiffOutCoefMax=[]  ReciprocalOutMin=[]  ReciprocalOutMax=[]  SumDenOutMin=[]  SumDenOutMax=[]  SumNumOutMin=[]  SumNumOutMax=[]  DivideOutMin=[]  DivideOutMax=[]  UdiffTsProdOutMin=[]  UdiffTsProdOutMax=[]  NTsProdOutMin=[]  NTsProdOutMax=[]  UintegralTsProdOutMin=[]  UintegralTsProdOutMax=[]  UngainTsProdOutMin=[]  UngainTsProdOutMax=[]  ClampingZeroOutDataTypeStr=Inherit: Inherit via back propagation  ClampingZeroOutMin=[]  ClampingZeroOutMax=[]  FilterDenConstantOutDataTypeStr=Inherit: Inherit via back propagation  FilterDenConstantOutMin=[]  FilterDenConstantOutMax=[]  PCopyOutDataTypeStr=Inherit: Inherit via back propagation  PCopyOutMin=[]  PCopyOutMax=[]  NCopyOutDataTypeStr=Inherit: Inherit via back propagation  NCopyOutMin=[]  NCopyOutMax=[]  IntegratorContinuousStateAttributes=''  IntegratorStateMustResolveToSignalObject=off  IntegratorRTWStateStorageClass=Auto  FilterContinuousStateAttributes=''  FilterStateMustResolveToSignalObject=off  FilterRTWStateStorageClass=Auto  ParallelPVariant=InternalParameters  IdealPVariant=Disabled  IVariant=InternalParameters  DVariant=Disabled  IntegratorVariant=Discrete  SatVariant=Enabled  AWVariant=Passthrough  PCopyVariant=Disabled  TRVariant=Disabled  FdbkBlocksVariant=Forward  IdealPFdbkVariant=Disabled  SatFdbkVariant=Disabled  DerivativeFilterVariant=Disabled  NVariant=Disabled  NCopyVariant=Disabled_SignalSpec  FilterICVariant=Disabled  IntegratorICVariant=InternalICs  ExternalResetVariant=Disabled  TRSumVariant=Passthrough  SumFdbkVariant=Disabled  SumVariant=Sum_PI  TsampFilterVariant=InternalTs  TsampNgainVariant=Passthrough  TsampIntegralVariant=Disabled_SignalSpec  ExternalSaturationOutDataTypeStr=Inherit: Same as second input  DerivativeSourceVariant=Disabled  PreIntVariant=InternalPreInt
  voltage controlled1 : slpidlib/PID Controller  Controller=PI  Form=Parallel  TimeDomain=Discrete-time  UseExternalTs=off  SampleTime=500e-6  IntegratorMethod=Forward Euler  FilterMethod=Forward Euler  ControllerParametersSource=internal  P=40  I=2000  UseKiTs=off  D=0  UseExternalDerivativeSource=off  N=100  UseFilter=on  TunerSelectOption=Transfer Function Based (PID Tuner App)  InitialConditionSource=internal  InitialConditionForIntegrator=0  InitialConditionForFilter=0  DifferentiatorICPrevScaledInput=0  ExternalReset=none  TrackingMode=off  Kt=1  LimitOutput=on  SatLimitsSource=internal  UpperSaturationLimit=22  LowerSaturationLimit=0  LinearizeAsGain=on  AntiWindupMode=none  Kb=1  LimitIntegrator=off  UpperIntegratorSaturationLimit=inf  LowerIntegratorSaturationLimit=-inf  POutMin=[]  POutMax=[]  IOutMin=[]  IOutMax=[]  DOutMin=[]  DOutMax=[]  NOutMin=[]  NOutMax=[]  SumOutMin=[]  SumOutMax=[]  SaturationOutMin=[]  SaturationOutMax=[]  PParamMin=[]  PParamMax=[]  IParamMin=[]  IParamMax=[]  DParamMin=[]  DParamMax=[]  NParamMin=[]  NParamMax=[]  KbParamMin=[]  KbParamMax=[]  KtParamMin=[]  KtParamMax=[]  KbOutMin=[]  KbOutMax=[]  KtOutMin=[]  KtOutMax=[]  IntegratorOutMin=[]  IntegratorOutMax=[]  FilterOutMin=[]  FilterOutMax=[]  SumI1OutMin=[]  SumI1OutMax=[]  SumI2OutMin=[]  SumI2OutMax=[]  SumI3OutMin=[]  SumI3OutMax=[]  SumI4OutMin=[]  SumI4OutMax=[]  SumDOutMin=[]  SumDOutMax=[]  DifferentiatorOutMin=[]  DifferentiatorOutMax=[]  FilterDiffOutCoefMin=[]  FilterDiffOutCoefMax=[]  ReciprocalOutMin=[]  ReciprocalOutMax=[]  SumDenOutMin=[]  SumDenOutMax=[]  SumNumOutMin=[]  SumNumOutMax=[]  DivideOutMin=[]  DivideOutMax=[]  UdiffTsProdOutMin=[]  UdiffTsProdOutMax=[]  NTsProdOutMin=[]  NTsProdOutMax=[]  UintegralTsProdOutMin=[]  UintegralTsProdOutMax=[]  UngainTsProdOutMin=[]  UngainTsProdOutMax=[]  ClampingZeroOutDataTypeStr=Inherit: Inherit via back propagation  ClampingZeroOutMin=[]  ClampingZeroOutMax=[]  FilterDenConstantOutDataTypeStr=Inherit: Inherit via back propagation  FilterDenConstantOutMin=[]  FilterDenConstantOutMax=[]  PCopyOutDataTypeStr=Inherit: Inherit via back propagation  PCopyOutMin=[]  PCopyOutMax=[]  NCopyOutDataTypeStr=Inherit: Inherit via back propagation  NCopyOutMin=[]  NCopyOutMax=[]  IntegratorContinuousStateAttributes=''  IntegratorStateMustResolveToSignalObject=off  IntegratorRTWStateStorageClass=Auto  FilterContinuousStateAttributes=''  FilterStateMustResolveToSignalObject=off  FilterRTWStateStorageClass=Auto  ParallelPVariant=InternalParameters  IdealPVariant=Disabled  IVariant=InternalParameters  DVariant=Disabled  IntegratorVariant=Discrete  SatVariant=Enabled  AWVariant=Passthrough  PCopyVariant=Disabled  TRVariant=Disabled  FdbkBlocksVariant=Forward  IdealPFdbkVariant=Disabled  SatFdbkVariant=Disabled  DerivativeFilterVariant=Disabled  NVariant=Disabled  NCopyVariant=Disabled_SignalSpec  FilterICVariant=Disabled  IntegratorICVariant=InternalICs  ExternalResetVariant=Disabled  TRSumVariant=Passthrough  SumFdbkVariant=Disabled  SumVariant=Sum_PI  TsampFilterVariant=InternalTs  TsampNgainVariant=Passthrough  TsampIntegralVariant=Disabled_SignalSpec  ExternalSaturationOutDataTypeStr=Inherit: Same as second input  DerivativeSourceVariant=Disabled  PreIntVariant=InternalPreInt
  disch_out+ : PMIOPort  Side=Left
  disch_out- : PMIOPort  Port=2  Side=Left
  charge_in+ : PMIOPort  Port=3  Side=Left
  charge_in- : PMIOPort  Port=4  Side=Left
  disch_in+ : PMIOPort  Port=5  Side=Right
  disch_in- : PMIOPort  Port=6  Side=Right
  charge_out+ : PMIOPort  Port=7  Side=Right
  charge_out- : PMIOPort  Port=8  Side=Right
  tag scope: Vload=global
  wires:
  [S_P1] -> Mosfet2/1
  Add5/1 -> voltage controlled1/1
  [S_N1] -> Mosfet3/1
  PWM Generator (DC-DC)3/1 -> NOT1/1, [S_P1]
  Gain2/1 -> [Ib_ref1]
  [S_N] -> Mosfet1/1
  [S_P] -> Mosfet/1
  Constant5/1 -> Add5/1
  Voltage Measurement1/1 -> [Vload]
  [Ib_ref1] -> Add4/2
  voltage controlled1/1 -> Gain2/1
  current controlled/1 -> PWM Generator (DC-DC)3/1
  Add4/1 -> current controlled/1
  NOT1/1 -> [S_N1]
  [Vb] -> Add5/2
  [Ib] -> Add4/1
  connections:
  Series RLC Branch5/RConn1 -- charge_in-/RConn1 -- Mosfet3/RConn1 -- charge_out-/RConn1 -- Series RLC Branch6/RConn1
  Mosfet3/LConn1 -- Mosfet2/RConn1 -- Series RLC Branch4/LConn1
  Series RLC Branch5/LConn1 -- charge_in+/RConn1 -- Mosfet2/LConn1
  Series RLC Branch3/LConn1 -- disch_out+/RConn1 -- Mosfet/LConn1 -- Voltage Measurement1/LConn1
  Series RLC Branch6/LConn1 -- charge_out+/RConn1 -- Series RLC Branch7/LConn1
  Series RLC Branch3/RConn1 -- Voltage Measurement1/LConn2 -- disch_out-/RConn1 -- Mosfet1/RConn1 -- disch_in-/RConn1 -- Series RLC Branch2/RConn1
  Series RLC Branch4/RConn1 -- Series RLC Branch7/RConn1
  Mosfet/RConn1 -- Series RLC Branch1/RConn1 -- Mosfet1/LConn1
  Series RLC Branch2/LConn1 -- disch_in+/RConn1 -- Series RLC Branch1/LConn1

== system IOT_Charger/MPPT and PV Controller/Battery controller/Battery Controller ==
  V_Dc : Inport
  370 : Inport  Port=2
  I_bt : Inport  Port=3
  Add : Sum
  Add1 : Sum  Inputs=+-|
  Add2 : Sum  Inputs=+-|
  Constant : Constant  Value=-1
  Demux5 : Demux  Outputs=2
  Gain : Gain  Gain=2
  PWM Generator (2-Level) : spsPWMGenerator2LevelLib/PWM Generator (2-Level)  ModulatorType=Single-phase half-bridge (2 pulses)  ModulatorMode=Unsynchronized  Fc=10000  Pc=90  nF=27  MinMax="[ -1  1 ]"  SamplingTechnique=Natural  ModulatingSignals=off  m=0.8  Freq=60  Phase=0  Ts=0  ShowCarrierOutport=off
  Saturation : Saturate  UpperLimit=370  LowerLimit=0
  Saturation1 : Saturate  UpperLimit=1  LowerLimit=0
  Transfer Fcn1 : TransferFcn  Denominator=[1e-4 1]
  Transfer Fcn2 : TransferFcn  Denominator=[1e-4 1]
  Transfer Fcn3 : TransferFcn  Denominator=[1e-4 1]
  Pulse 1 : Outport  OutputWhenDisabled=reset  InitialOutput=0  VectorParamsAs1DForOutWhenUnconnected=off
  Pulse 2 : Outport  Port=2  OutputWhenDisabled=reset  InitialOutput=0  VectorParamsAs1DForOutWhenUnconnected=off
  wires:
  370/1 -> Saturation/1  "Vref"
  Add/1 -> PWM Generator (2-Level)/1  "duty_to_-1_1"
  Gain/1 -> Add/1
  Constant/1 -> Add/2
  Saturation/1 -> Add1/2  "Vref"
  V_Dc/1 -> Add1/1
  Add1/1 -> Transfer Fcn1/1  "err"
  I_bt/1 -> Add2/1
  Add2/1 -> Transfer Fcn2/1  "err"
  Transfer Fcn1/1 -> Transfer Fcn3/1  "Err_filter"
  Transfer Fcn2/1 -> Saturation1/1  "err_filter"
  Transfer Fcn3/1 -> Add2/2
  Saturation1/1 -> Gain/1
  Demux5/1 -> Pulse 1/1
  Demux5/2 -> Pulse 2/1
  PWM Generator (2-Level)/1 -> Demux5/1

== system IOT_Charger/MPPT and PV Controller/Battery controller/PWM Controller 2 ==
  Vdc : Inport
  Enable : EnablePort  StatesWhenEnabling=reset
  Add : Sum
  Constant : Constant  Value=200*sqrt(2)
  Constant1 : Constant  Value=1e-6
  Divide : Product  Inputs=*/
  PWM Generator (2-Level) : spsPWMGenerator2LevelLib/PWM Generator (2-Level)  ModulatorType=Single-phase full-bridge (4 pulses)  ModulatorMode=Unsynchronized  Fc=10000  Pc=90  nF=27  MinMax="[ -1  1 ]"  SamplingTechnique=Natural  ModulatingSignals=off  m=0.8  Freq=60  Phase=0  Ts=0  ShowCarrierOutport=off
  Product2 : Product  RndMeth=Zero  SampleTime=5e-6
  Uref Generation (60Hz) : Sin  Frequency=2*pi*60  SampleTime=5e-6
  Pulse : Outport  OutputWhenDisabled=reset  InitialOutput=[0 0 0 0]  VectorParamsAs1DForOutWhenUnconnected=off
  wires:
  PWM Generator (2-Level)/1 -> Pulse/1
  Product2/1 -> PWM Generator (2-Level)/1
  Uref Generation (60Hz)/1 -> Product2/2
  Divide/1 -> Product2/1
  Vdc/1 -> Add/1
  Constant/1 -> Divide/1
  Constant1/1 -> Add/2
  Add/1 -> Divide/2

== system IOT_Charger/MPPT and PV Controller/Inverter controller/Inverter Controller ==
  V_Dc : Inport
  370 : Inport  Port=2
  V_Sys_Secondary : Inport  Port=3
  I_Sys_Secondary : Inport  Port=4
  Enable : EnablePort  StatesWhenEnabling=reset
  Add : Sum
  Add1 : Sum  Inputs=+-|
  Add2 : Sum  Inputs=+-|
  Constant : Constant  Value=-1
  Constant4 : Constant
  Divide1 : Product  Inputs=*/
  Gain : Gain  Gain=2
  PLL : spsPLLLib/PLL  Fmin=45  Par_Init=[0, 60]  ParK=[180, 3200, 1]  TcD=1e-4  MaxRateChangeFreq=12  FilterCutOffFreq=25  Ts=0  AGC=on
      settings: LibrarySourceBlock=sps_lib/Control/PLL
  PWM Generator (2-Level) : spsPWMGenerator2LevelLib/PWM Generator (2-Level)  ModulatorType=Single-phase full-bridge (4 pulses)  ModulatorMode=Unsynchronized  Fc=10000  Pc=90  nF=27  MinMax="[ -1  1 ]"  SamplingTechnique=Natural  ModulatingSignals=off  m=0.8  Freq=60  Phase=0  Ts=0  ShowCarrierOutport=off
  Product1 : Product  RndMeth=Zero
  Saturation1 : Saturate  UpperLimit=1  LowerLimit=-1
  Saturation3 : Saturate  UpperLimit=50  LowerLimit=-50
  Terminator : Terminator
  Transfer Fcn1 : TransferFcn  Denominator=[1e-4 1]
  Transfer Fcn2 : TransferFcn  Denominator=[1e-4 1]
  Transfer Fcn3 : TransferFcn  Denominator=[1e-4 1]
  Trigonometric Function : Trigonometry
  Pulse : Outport  OutputWhenDisabled=reset  InitialOutput=[0 0 0 0]  VectorParamsAs1DForOutWhenUnconnected=off
  wires:
  PWM Generator (2-Level)/1 -> Pulse/1
  370/1 -> Add1/2  "Vref"
  Add/1 -> PWM Generator (2-Level)/1  "duty_to_-1_1"
  Gain/1 -> Add/1
  Constant/1 -> Add/2
  V_Dc/1 -> Add1/1
  Add1/1 -> Transfer Fcn1/1  "err"
  I_Sys_Secondary/1 -> Add2/1
  Add2/1 -> Transfer Fcn2/1  "err"
  Transfer Fcn2/1 -> Saturation1/1  "err_filter"
  Transfer Fcn1/1 -> Saturation3/1  "Iref"
  Product1/1 -> Transfer Fcn3/1
  Saturation1/1 -> Gain/1
  Divide1/1 -> PLL/1  "V_Sys_Secondary"
  PLL/2 -> Trigonometric Function/1  "wt"
  Constant4/1 -> Divide1/2
  V_Sys_Secondary/1 -> Divide1/1
  Transfer Fcn3/1 -> Add2/2
  Saturation3/1 -> Product1/1
  Trigonometric Function/1 -> Product1/2
  PLL/1 -> Terminator/1  "Freq"

== system IOT_Charger/MPPT and PV Controller/MMPT Controller/PV Controller ==
  V_pv : Inport
  I_pv : Inport  Port=2
  Vref : Inport  Port=3
  Add3 : Sum
  Add4 : Sum  Inputs=+-|
  Add5 : Sum  Inputs=+-|
  Add6 : Sum  Inputs=+-|
  Constant3 : Constant  Value=-1
  Constant5 : Constant
  Demux2 : Demux  Outputs=2
  Gain2 : Gain  Gain=2
  PWM Generator (2-Level) : spsPWMGenerator2LevelLib/PWM Generator (2-Level)  ModulatorType=Single-phase full-bridge (4 pulses)  ModulatorMode=Unsynchronized  Fc=10000  Pc=90  nF=27  MinMax="[ -1  1 ]"  SamplingTechnique=Natural  ModulatingSignals=off  m=0.8  Freq=60  Phase=0  Ts=0  ShowCarrierOutport=off
  Saturation2 : Saturate  UpperLimit=280  LowerLimit=0
  Saturation3 : Saturate  UpperLimit=1  LowerLimit=0
  Terminator1 : Terminator
  Transfer Fcn5 : TransferFcn  Denominator=[1e-4 1]
  Transfer Fcn6 : TransferFcn  Denominator=[1e-4 1]
  Pulse : Outport  VectorParamsAs1DForOutWhenUnconnected=off
  wires:
  PWM Generator (2-Level)/1 -> Demux2/1
  Vref/1 -> Saturation2/1
  I_pv/1 -> Add5/1
  Add3/1 -> PWM Generator (2-Level)/1  "duty_to_-1_1"
  Gain2/1 -> Add3/1
  Constant3/1 -> Add3/2
  Demux2/2 -> Terminator1/1
  Saturation2/1 -> Add4/2  "Vref"
  Add4/1 -> Transfer Fcn5/1  "err"
  Add5/1 -> Transfer Fcn6/1  "err"
  Transfer Fcn6/1 -> Saturation3/1
  Saturation3/1 -> Add6/2
  Constant5/1 -> Add6/1
  Add6/1 -> Gain2/1
  Transfer Fcn5/1 -> Add5/2  "Err_filter"
  V_pv/1 -> Add4/1
  Demux2/1 -> Pulse/1

== system IOT_Charger/Vechicle BMS Monitoring/BMS Discharge/Function logic block ==
  Terminal voltage : Inport
  Current : Inport  Port=2
  Temperature : Inport  Port=3
  Display : Display
  Display1 : Display
  Display2 : Display
  Max Temp : Constant  Value=333
  Min temp : Constant  Value=253
  OR : Logic  Operator=OR  AllPortsSameDT=off  OutDataTypeStr=boolean
  OR1 : Logic  Operator=OR  Inputs=3  AllPortsSameDT=off  OutDataTypeStr=boolean
  Over current : Constant  Value=155
  Relational Operator : RelationalOperator  Operator=<=  OutDataTypeStr=boolean  RndMeth=Simplest  InputSameDT=off
  Relational Operator1 : RelationalOperator  OutDataTypeStr=boolean  RndMeth=Simplest  InputSameDT=off
  Relational Operator2 : RelationalOperator  OutDataTypeStr=boolean  RndMeth=Simplest  InputSameDT=off
  Relational Operator3 : RelationalOperator  OutDataTypeStr=boolean  RndMeth=Simplest  InputSameDT=off
  Under voltage : Constant  Value=2.7
  Discharge Terget : Outport
  wires:
  Terminal voltage/1 -> Relational Operator/1
  Under voltage/1 -> Relational Operator/2
  Over current/1 -> Relational Operator1/2
  Current/1 -> Relational Operator1/1
  Temperature/1 -> Relational Operator3/1, Relational Operator2/1
  Max Temp/1 -> Relational Operator2/2
  Min temp/1 -> Relational Operator3/2
  Relational Operator2/1 -> OR/1
  Relational Operator3/1 -> OR/2
  OR/1 -> Display2/1, OR1/3
  Relational Operator1/1 -> Display1/1, OR1/2
  Relational Operator/1 -> Display/1, OR1/1
  OR1/1 -> Discharge Terget/1

== system IOT_Charger/Vechicle BMS Monitoring1/BMS Discharge/Function logic block ==
  Terminal voltage : Inport
  Current : Inport  Port=2
  Temperature : Inport  Port=3
  Display : Display
  Display1 : Display
  Display2 : Display
  Max Temp : Constant  Value=333
  Min temp : Constant  Value=253
  OR : Logic  Operator=OR  AllPortsSameDT=off  OutDataTypeStr=boolean
  OR1 : Logic  Operator=OR  Inputs=3  AllPortsSameDT=off  OutDataTypeStr=boolean
  Over current : Constant  Value=155
  Relational Operator : RelationalOperator  Operator=<=  OutDataTypeStr=boolean  RndMeth=Simplest  InputSameDT=off
  Relational Operator1 : RelationalOperator  OutDataTypeStr=boolean  RndMeth=Simplest  InputSameDT=off
  Relational Operator2 : RelationalOperator  OutDataTypeStr=boolean  RndMeth=Simplest  InputSameDT=off
  Relational Operator3 : RelationalOperator  OutDataTypeStr=boolean  RndMeth=Simplest  InputSameDT=off
  Under voltage : Constant  Value=2.7
  Discharge Terget : Outport
  wires:
  Terminal voltage/1 -> Relational Operator/1
  Under voltage/1 -> Relational Operator/2
  Over current/1 -> Relational Operator1/2
  Current/1 -> Relational Operator1/1
  Temperature/1 -> Relational Operator3/1, Relational Operator2/1
  Max Temp/1 -> Relational Operator2/2
  Min temp/1 -> Relational Operator3/2
  Relational Operator2/1 -> OR/1
  Relational Operator3/1 -> OR/2
  OR/1 -> Display2/1, OR1/3
  Relational Operator1/1 -> Display1/1, OR1/2
  Relational Operator/1 -> Display/1, OR1/1
  OR1/1 -> Discharge Terget/1
